simulink model "sim_df2"  (Simulink 3.00)
settings: Solver=ode45  SolverMode=SingleTasking  StartTime=0  StopTime=tf  MaxStep=maxstep  RelTol=tol  AbsTol=tol
values from neighbouring files (symbols this model uses):
  endPt = [Xshoulder2motor Yshoulder2motor]         -trialData(trial,4:5)    [doSim.m]
  ICs = [qI(1,2) 0; qI(1,3) 0]    [doSim.m]
undefined symbols (not defined in the file or in its folder): Bact, Kact, speedThresh
settings Model: SaveTime=off  SaveOutput=off  LastModifiedBy=patton

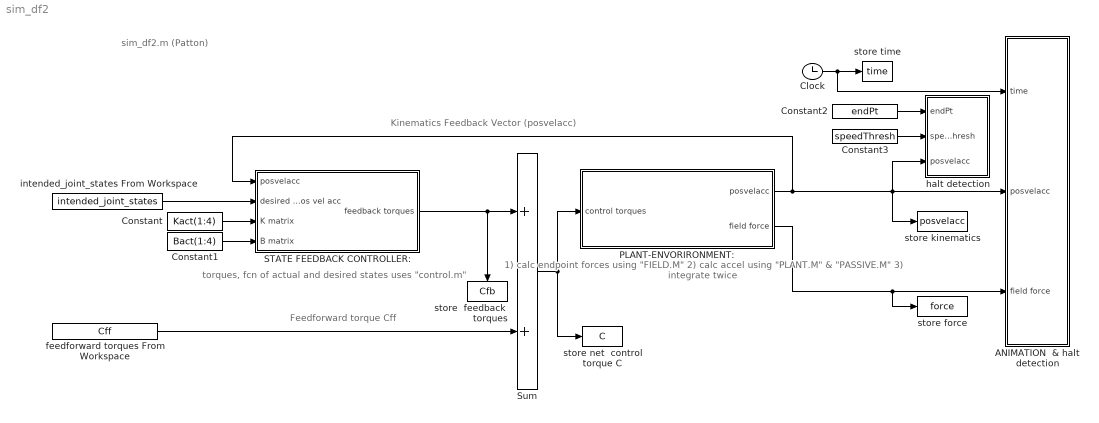
== system sim_df2 ==
  note: sim_df2.m (Patton)
  note: Kinematics Feedback Vector (posvelacc)
  note: 1) calc endpoint forces using "FIELD.M"
      | 2) calc accel using "PLANT.M" & "PASSIVE.M"
      | 3) integrate twice
  note: torques, fcn of actual and
      | desired states uses "control.m"
  note: Feedforward torque Cff
  ANIMATION  & halt detection : Subsystem
  Clock : Clock
      settings: DisplayTime=off  Decimation=10
  Constant : Constant  Value=Kact(1:4)
  Constant1 : Constant  Value=Bact(1:4)
  Constant2 : Constant  Value=endPt
  Constant3 : Constant  Value=speedThresh
  PLANT-ENVORIRONMENT: : Subsystem
  STATE FEEDBACK CONTROLLER: : Subsystem
  Sum : Sum  Inputs=++  SaturateOnIntegerOverflow=on
  feedforward torques From Workspace : FromWorkspace  VariableName=Cff  SampleTime=0  HoldFinalValue=off
  halt detection : Subsystem
  intended_joint_states From Workspace : FromWorkspace  VariableName=intended_joint_states  SampleTime=0  HoldFinalValue=off
  store  feedback  torques : ToWorkspace  VariableName=Cfb  SampleTime=0  SaveFormat=Matrix
      settings: Orientation=down  Buffer=10000
  store force : ToWorkspace  VariableName=force  SampleTime=0  SaveFormat=Matrix
      settings: Buffer=10000
  "store kinematics " : ToWorkspace  VariableName=posvelacc  SampleTime=0  SaveFormat=Matrix
      settings: Buffer=10000
  store net  control torque C : ToWorkspace  VariableName=C  SampleTime=0  SaveFormat=Matrix
      settings: Buffer=10000
  store time : ToWorkspace  VariableName=time  SampleTime=0  SaveFormat=Matrix
      settings: Buffer=10000
  wires:
  feedforward torques From Workspace/1 -> Sum/2
  Sum/1 -> PLANT-ENVORIRONMENT:/1(control torques), store net  control torque C/1
  PLANT-ENVORIRONMENT:/1(posvelacc) -> STATE FEEDBACK CONTROLLER:/1(posvelacc), ANIMATION  & halt detection/2(posvelacc), "store kinematics "/1, halt detection/3(posvelacc)
  Constant/1 -> STATE FEEDBACK CONTROLLER:/3(K matrix)
  Constant1/1 -> STATE FEEDBACK CONTROLLER:/4(B matrix)
  intended_joint_states From Workspace/1 -> STATE FEEDBACK CONTROLLER:/2(desired pos vel acc)
  STATE FEEDBACK CONTROLLER:/1(feedback torques) -> Sum/1, store  feedback  torques/1
  Constant2/1 -> halt detection/1(endPt)
  Constant3/1 -> halt detection/2(speedThresh)
  Clock/1 -> store time/1, ANIMATION  & halt detection/1(time)
  PLANT-ENVORIRONMENT:/2(field force) -> ANIMATION  & halt detection/3(field force), store force/1

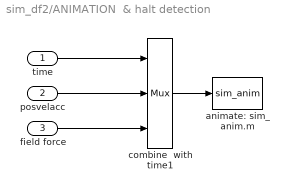
== system sim_df2/ANIMATION  & halt detection ==
  time : Inport  Port=1  PortWidth=-1  SampleTime=-1  DataType=auto
      settings: SignalType=auto
  posvelacc : Inport  Port=2  PortWidth=-1  SampleTime=-1  DataType=auto
      settings: SignalType=auto
  field force : Inport  Port=3  PortWidth=-1  SampleTime=-1  DataType=auto
      settings: SignalType=auto
  animate: sim_anim.m : MATLABFcn  MATLABFcn=sim_anim  OutputWidth=0  OutputSignalType=auto
  combine  with time1 : Mux  Inputs=3
      settings: DisplayOption=none
  wires:
  combine  with time1/1 -> animate: sim_anim.m/1
  time/1 -> combine  with time1/1
  field force/1 -> combine  with time1/3
  posvelacc/1 -> combine  with time1/2

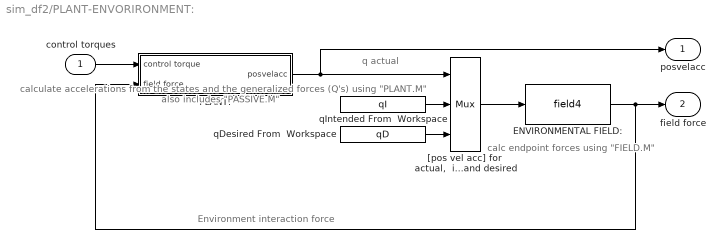
== system sim_df2/PLANT-ENVORIRONMENT: ==
  note: Environment interaction force
  note: q actual
  note: calculate accelerations from the states and
      | the generalized forces (Q's) using "PLANT.M"
      | also includes "PASSIVE.M"
  note: calc endpoint forces
      | using "FIELD.M"
  control torques : Inport  Port=1  PortWidth=-1  SampleTime=-1  DataType=auto
      settings: SignalType=auto
  ENVIRONMENTAL FIELD: : MATLABFcn  MATLABFcn=field4  OutputWidth=2  OutputSignalType=auto
  PLANT: : Subsystem
  "[pos vel acc] for  actual,  intended,  and desired" : Mux  Inputs=3
      settings: DisplayOption=none
  qDesired From  Workspace : FromWorkspace  VariableName=qD  SampleTime=0  HoldFinalValue=off
  qIntended From  Workspace : FromWorkspace  VariableName=qI  SampleTime=0  HoldFinalValue=off
  posvelacc : Outport  Port=1  InitialOutput=0
  field force : Outport  Port=2  InitialOutput=0
  wires:
  control torques/1 -> PLANT:/1(control torque)
  "[pos vel acc] for  actual,  intended,  and desired"/1 -> ENVIRONMENTAL FIELD:/1
  PLANT:/1(" posvelacc") -> "[pos vel acc] for  actual,  intended,  and desired"/1, posvelacc/1
  qDesired From  Workspace/1 -> "[pos vel acc] for  actual,  intended,  and desired"/3
  qIntended From  Workspace/1 -> "[pos vel acc] for  actual,  intended,  and desired"/2
  ENVIRONMENTAL FIELD:/1 -> PLANT:/2(field force), field force/1

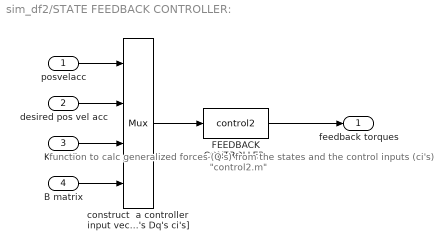
== system sim_df2/STATE FEEDBACK CONTROLLER: ==
  note: function to calc
      | generalized forces
      | (Q's) from the states
      | and the control
      | inputs (ci's)
      | "control2.m"
  posvelacc : Inport  Port=1  PortWidth=-1  SampleTime=-1  DataType=auto
      settings: SignalType=auto
  desired pos vel acc : Inport  Port=2  PortWidth=-1  SampleTime=-1  DataType=auto
      settings: SignalType=auto
  K matrix : Inport  Port=3  PortWidth=-1  SampleTime=-1  DataType=auto
      settings: SignalType=auto
  B matrix : Inport  Port=4  PortWidth=-1  SampleTime=-1  DataType=auto
      settings: SignalType=auto
  FEEDBACK CONTROLLER: : MATLABFcn  MATLABFcn=control2  OutputWidth=2  OutputSignalType=auto
  construct  a controller  input vector: [q's Dq's ci's] : Mux  Inputs=4
      settings: DisplayOption=none
  feedback torques : Outport  Port=1  InitialOutput=0
  wires:
  construct  a controller  input vector: [q's Dq's ci's]/1 -> FEEDBACK CONTROLLER:/1
  posvelacc/1 -> construct  a controller  input vector: [q's Dq's ci's]/1
  desired pos vel acc/1 -> construct  a controller  input vector: [q's Dq's ci's]/2
  K matrix/1 -> construct  a controller  input vector: [q's Dq's ci's]/3
  B matrix/1 -> construct  a controller  input vector: [q's Dq's ci's]/4
  FEEDBACK CONTROLLER:/1 -> feedback torques/1

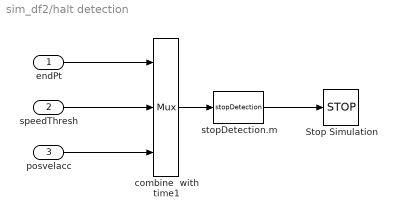
== system sim_df2/halt detection ==
  endPt : Inport  Port=1  PortWidth=-1  SampleTime=-1  DataType=auto
      settings: SignalType=auto
  speedThresh : Inport  Port=2  PortWidth=-1  SampleTime=-1  DataType=auto
      settings: SignalType=auto
  posvelacc : Inport  Port=3  PortWidth=-1  SampleTime=-1  DataType=auto
      settings: SignalType=auto
  Stop Simulation : Stop
  combine  with time1 : Mux  Inputs=3
      settings: DisplayOption=none
  stopDetection.m : MATLABFcn  MATLABFcn=stopDetection  OutputWidth=1  OutputSignalType=auto
  wires:
  stopDetection.m/1 -> Stop Simulation/1
  combine  with time1/1 -> stopDetection.m/1
  posvelacc/1 -> combine  with time1/3
  endPt/1 -> combine  with time1/1
  speedThresh/1 -> combine  with time1/2

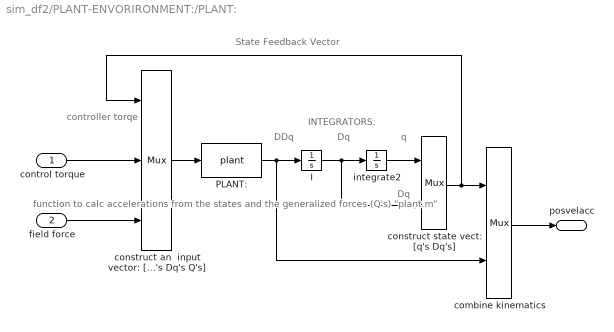
== system sim_df2/PLANT-ENVORIRONMENT:/PLANT: ==
  note: DDq
  note: Dq
  note: q
  note: Dq
  note: INTEGRATORS:
  note: State Feedback Vector
  note: controller
      | torqe
  note: function to calc
      | accelerations
      | from the states
      | and the
      | generalized
      | forces
      | (Q's)
      | "plant.m"
  control torque : Inport  Port=1  PortWidth=-1  SampleTime=-1  DataType=auto
      settings: SignalType=auto
  field force : Inport  Port=2  PortWidth=-1  SampleTime=-1  DataType=auto
      settings: SignalType=auto
  I : Integrator  ExternalReset=none  InitialConditionSource=internal  InitialCondition=ICs(:,2)  LimitOutput=off  UpperSaturationLimit=inf  LowerSaturationLimit=-inf  ShowSaturationPort=off  ShowStatePort=off  AbsoluteTolerance=auto
  PLANT: : MATLABFcn  MATLABFcn=plant  OutputWidth=2  OutputSignalType=auto
  combine kinematics : Mux  Inputs=2
      settings: DisplayOption=none
  construct an  input vector: [q's Dq's Q's] : Mux  Inputs=3
      settings: DisplayOption=none
  construct state vect: [q's Dq's] : Mux  Inputs=2
      settings: DisplayOption=none
  integrate2 : Integrator  ExternalReset=none  InitialConditionSource=internal  InitialCondition=ICs(:,1)  LimitOutput=off  UpperSaturationLimit=inf  LowerSaturationLimit=-inf  ShowSaturationPort=off  ShowStatePort=off  AbsoluteTolerance=auto
  " posvelacc" : Outport  Port=1  InitialOutput=0
  wires:
  control torque/1 -> construct an  input vector: [q's Dq's Q's]/2
  construct an  input vector: [q's Dq's Q's]/1 -> PLANT:/1
  integrate2/1 -> construct state vect: [q's Dq's]/1
  I/1 -> integrate2/1, construct state vect: [q's Dq's]/2
  PLANT:/1 -> I/1, combine kinematics/2
  construct state vect: [q's Dq's]/1 -> combine kinematics/1, construct an  input vector: [q's Dq's Q's]/1
  combine kinematics/1 -> " posvelacc"/1
  field force/1 -> construct an  input vector: [q's Dq's Q's]/3
